simulink model "Child"  (R2023a)
settings: Solver=FixedStepAuto  StartTime=0.0  StopTime=inf  RelTol=1e-3
libraries: androiduilib x5, androidcommunicationlib x4, androidaudiovideolib x3, androidsensorlib x3
settings Model: Creator=Abhishek  LastModifiedBy=aashm
settings OptimizationCC: EnhancedBackFolding=on  PassReuseOutputArgsThreshold=0  MaxStackSize=64  OptimizeBlockOrder=speed  DifferentSizesBufferReuse=on  OptimizationCustomize=off
settings DebuggingCC: ParameterTunabilityLossMsg=error
settings HardwareCC: ProdBitPerPointer=32  ProdBitPerSizeT=32  ProdBitPerPtrDiffT=32  ProdLargestAtomicInteger=Long  ProdLargestAtomicFloat=Double  ProdWordSize=32  ProdHWDeviceType=ARM Compatible->ARM Cortex  UseEmbeddedCoderFeatures=off  UseSimulinkCoderFeatures=off
settings SFSimCC: MATLABDynamicMemAlloc=off
settings RTWCC: Description=Embedded Coder  SystemTargetFile=ert.tlc  HardwareBoard=Android Device  TLCOptions="-aInlineSetEventsForThisBaseRateFcn=TLC_FALSE -aSuppressMultiTaskScheduler=TLC_FALSE  -aRateBasedStepFcn=0"  TemplateMakefile=ert_default_tmf  RTWVerbose=off  Toolchain=Android SDK/NDK Tools
settings CodeAppCC: ForceParamTrailComments=on  OperatorAnnotations=on
settings ERTTargetCC: ERTCustomFileBanners=off  SupportContinuousTime=on  SupportNonInlinedSFcns=on  RemoveResetFunc=off  ModelStepFunctionPrototypeControlCompliant=off

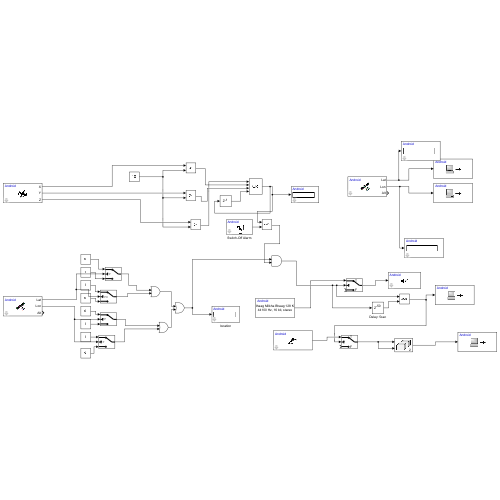
[thumbnail: Simulink's stored preview of the top-level diagram]
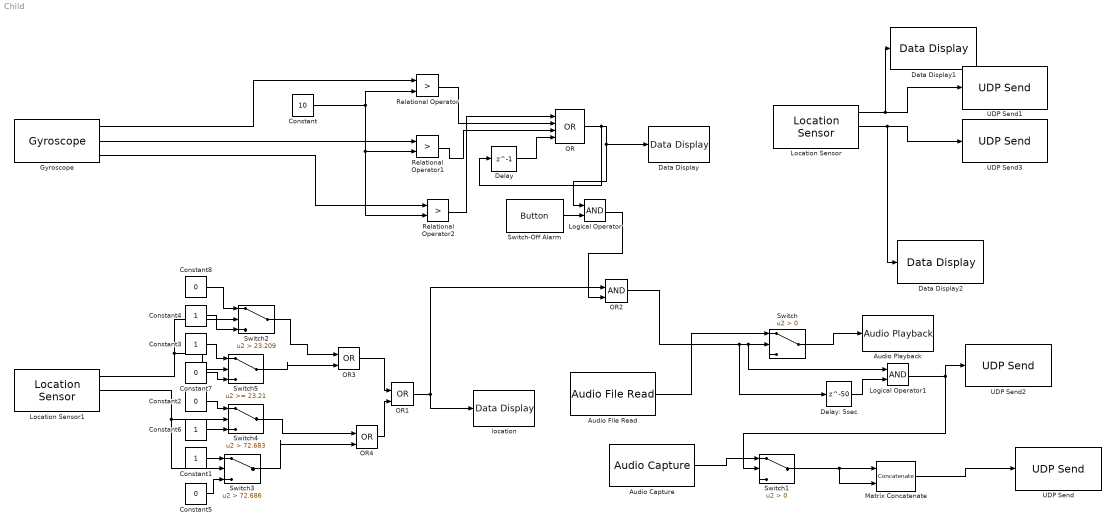
== system Child ==
  Audio Capture : androidaudiovideolib/Audio Capture  SampleFreq=24000  FrameSize=2400  SampleTime=0.1  SimulateUsing=Code generation  DeviceStr=0  QueueDuration=0  BlockPlatform=Android  AudioSamplingFreq=44100
  Audio File Read : androidaudiovideolib/Audio File Read  FileName=C:\Users\aashm\Music\Zinda - Bhaag Milkha Bhaag 128 Kbps.mp3  FrameSize=4410
  Audio Playback : androidaudiovideolib/Audio Playback  SampleFreq=44100  AudioSamplingFreq=44100  SampleTime=0.1  DeviceStr=0  QueueDuration=0  BlockPlatform=Android
  Constant : Constant  Value=10
  Constant{1,3..4,6} (4 alike) : Constant
  Constant{2,5,7..8} (4 alike) : Constant  Value=0
  Data Display : androiduilib/Data Display  DataDisplayId=Child/Data_Display  Format=Float  Precision=6  SimulateUsing=Code generation  blockPlatform=Android
  Data Display1 : androiduilib/Data Display  DataDisplayId=Child/Data_Display1  Format=Float  Precision=6  SimulateUsing=Code generation  blockPlatform=Android
  Data Display2 : androiduilib/Data Display  DataDisplayId=Child/Data_Display2  Format=Float  Precision=6  SimulateUsing=Code generation  blockPlatform=Android
  Delay : Delay  DelayLength=1
  Delay: 5sec : Delay  DelayLength=50  InitialCondition=0
  Gyroscope : androidsensorlib/Gyroscope  OutputVector=off  SampleTime=0.1  BlockPlatform=Android
  Location Sensor : androidsensorlib/Location Sensor  OutputVector=off  SampleTime=0.1  BlockPlatform=Android
  Location Sensor1 : androidsensorlib/Location Sensor  OutputVector=off  SampleTime=0.1  BlockPlatform=Android
  Logical Operator : Logic  AllPortsSameDT=off  OutDataTypeStr=boolean
  Logical Operator1 : Logic  AllPortsSameDT=off  OutDataTypeStr=boolean
  Matrix Concatenate : Concatenate  Mode=Multidimensional array  ConcatenateDimension=2
  OR : Logic  Operator=OR  Inputs=4  AllPortsSameDT=off  OutDataTypeStr=boolean
  OR1 : Logic  Operator=OR  IconShape=distinctive  AllPortsSameDT=off  OutDataTypeStr=boolean
  OR2 : Logic  IconShape=distinctive  AllPortsSameDT=off  OutDataTypeStr=boolean
  OR3 : Logic  Operator=OR  IconShape=distinctive  AllPortsSameDT=off  OutDataTypeStr=boolean
  OR4 : Logic  Operator=OR  IconShape=distinctive  AllPortsSameDT=off  OutDataTypeStr=boolean
  Relational Operator : RelationalOperator  Operator=>  OutDataTypeStr=boolean  RndMeth=Simplest  InputSameDT=off
  Relational Operator1 : RelationalOperator  Operator=>  OutDataTypeStr=boolean  RndMeth=Simplest  InputSameDT=off
  Relational Operator2 : RelationalOperator  Operator=>  OutDataTypeStr=boolean  RndMeth=Simplest  InputSameDT=off
  Switch : Switch  Criteria=u2 > Threshold  SaturateOnIntegerOverflow=off  InputSameDT=off
  Switch-Off Alarm : androiduilib/Button  ButtonState=Pressed  ButtonId=Child/Switch-Off_Alarm  State=on  SampleTime=0.1  BlockPlatform=Android
  Switch1 : Switch  Criteria=u2 > Threshold  SaturateOnIntegerOverflow=off  InputSameDT=off
  Switch2 : Switch  Criteria=u2 > Threshold  Threshold=23.209  SaturateOnIntegerOverflow=off  InputSameDT=off
  Switch3 : Switch  Criteria=u2 > Threshold  Threshold=72.686  SaturateOnIntegerOverflow=off  InputSameDT=off
  Switch4 : Switch  Criteria=u2 > Threshold  Threshold=72.683  SaturateOnIntegerOverflow=off  InputSameDT=off
  Switch5 : Switch  Threshold=23.21  SaturateOnIntegerOverflow=off  InputSameDT=off
  UDP Send : androidcommunicationlib/UDP Send  remoteURL='10.7.62.98'  remotePort=25111  localURL='0.0.0.0'  localPortSource=Automatically determine  localPort=-1  sampletime=-1  blockPlatform=Android  separateLengthPort=0
  UDP Send1 : androidcommunicationlib/UDP Send  remoteURL='10.7.62.98'  remotePort=25114  localURL='0.0.0.0'  localPortSource=Automatically determine  localPort=-1  sampletime=-1  blockPlatform=Android  separateLengthPort=0
  UDP Send2 : androidcommunicationlib/UDP Send  remoteURL='10.7.62.98'  remotePort=25112  localURL='0.0.0.0'  localPortSource=Automatically determine  localPort=-1  sampletime=-1  blockPlatform=Android  separateLengthPort=0
  UDP Send3 : androidcommunicationlib/UDP Send  remoteURL='10.7.62.98'  remotePort=25113  localURL='0.0.0.0'  localPortSource=Automatically determine  localPort=-1  sampletime=-1  blockPlatform=Android  separateLengthPort=0
  location : androiduilib/Data Display  DataDisplayId=Child/location  Format=Float  Precision=6  SimulateUsing=Code generation  blockPlatform=Android
  wires:
  Gyroscope/1 -> Relational Operator/1
  Gyroscope/2 -> Relational Operator1/1
  Gyroscope/3 -> Relational Operator2/1
  Relational Operator1/1 -> OR/3
  OR/1 -> Delay/1, Logical Operator/1, Data Display/1
  Constant/1 -> Relational Operator2/2, Relational Operator1/2, Relational Operator/2
  Switch/1 -> Audio Playback/1
  Audio File Read/1 -> Switch/1
  Switch-Off Alarm/1 -> Logical Operator/2
  Relational Operator/1 -> OR/2
  Delay: 5sec/1 -> Logical Operator1/2
  Audio Capture/1 -> Switch1/1
  Logical Operator1/1 -> UDP Send2/1, Switch1/2
  Logical Operator/1 -> OR2/2
  Relational Operator2/1 -> OR/1
  Delay/1 -> OR/4
  Switch1/1 -> Matrix Concatenate/2, Matrix Concatenate/1
  Matrix Concatenate/1 -> UDP Send/1
  Location Sensor/1 -> Data Display1/1, UDP Send1/1
  Location Sensor/2 -> Data Display2/1, UDP Send3/1
  Constant3/1 -> Switch5/1
  Constant4/1 -> Switch2/3
  Constant5/1 -> Switch3/3
  Constant8/1 -> Switch2/1
  Location Sensor1/2 -> Switch4/2, Switch3/2
  Constant2/1 -> Switch4/1
  Constant7/1 -> Switch5/3
  Constant1/1 -> Switch3/1
  Location Sensor1/1 -> Switch5/2, Switch2/2
  Constant6/1 -> Switch4/3
  OR1/1 -> location/1, OR2/1
  OR2/1 -> Delay: 5sec/1, Logical Operator1/1, Switch/2
  Switch2/1 -> OR3/1
  Switch5/1 -> OR3/2
  Switch4/1 -> OR4/1
  Switch3/1 -> OR4/2
  OR3/1 -> OR1/1
  OR4/1 -> OR1/2
